simulink model "Simulink_Simulation"  (Simulink 10.1)
settings: Solver=ode23tb  StartTime=0.0  StopTime=3  RelTol=1e-3  EnableMultiTasking=on
undefined symbols (not defined in the file or in its folder): sigbuilder_block
libraries: powerlib x9, powerlib_meascontrol x1
settings Model: Creator=asus1  LastModifiedBy=x64
settings DataIOCC: LimitDataPoints=on
settings DebuggingCC: UnderspecifiedInitializationDetection=Simplified  MergeDetectMultiDrivingBlocksExec=error  SolverPrmCheckMsg=warning
settings GRTTargetCC: CombineOutputUpdateFcns=on  GRTInterface=off
settings ConfigComp: CovSFcnEnable=off
settings SimscapeCC: SimscapeNormalizeSystem=off

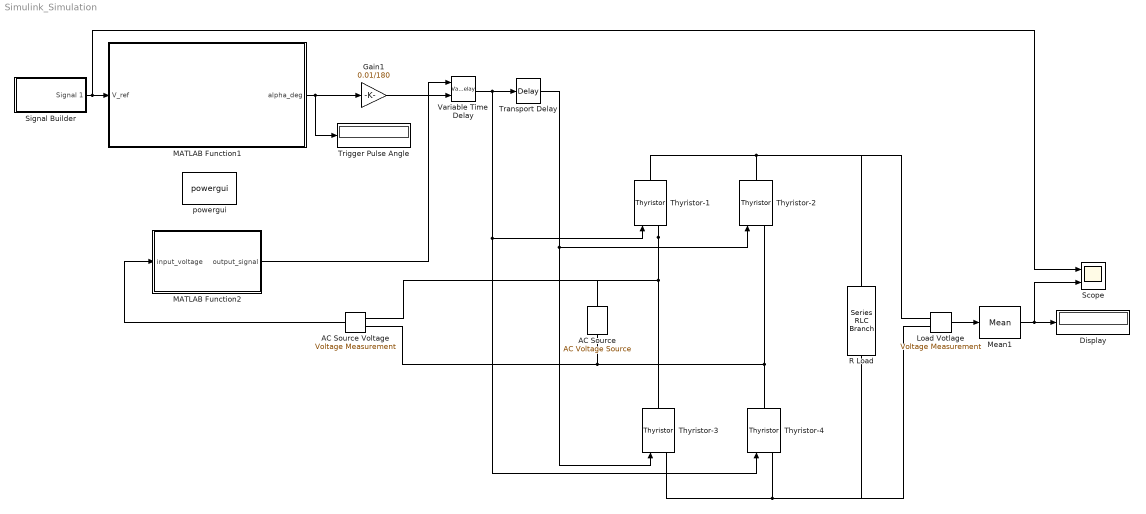
== system Simulink_Simulation ==
  AC Source : powerlib/Electrical Sources/AC Voltage Source  Amplitude=220*sqrt(2)  Phase=0  Frequency=50  SampleTime=0  Measurements=None  BusType=swing  Pref=10e3  Qref=0  Qmin=-inf  Qmax=+inf
  AC Source Voltage : powerlib/Measurements/Voltage Measurement  PhasorSimulation=off  OutputType=Complex  PSBequivalent=0
  "Display " : Display
  Gain1 : Gain  Gain=0.01/180
  Load Votlage : powerlib/Measurements/Voltage Measurement  PhasorSimulation=off  OutputType=Complex  PSBequivalent=0
  MATLAB Function1 : MATLAB Function  TreatAsAtomicUnit=on
  MATLAB Function2 : MATLAB Function  TreatAsAtomicUnit=on
  Mean1 : powerlib_meascontrol/Measurements/Mean  Freq=50  Vinit=0  Ts=0
  R Load : powerlib/Elements/Series RLC Branch  LConnTagsString=__new0  RConnTagsString=__new0  BranchType=R  Resistance=10  Inductance=1e-3  SetiL0=off  InitialCurrent=0  Capacitance=1e-6  Setx0=off  InitialVoltage=0  Measurements=None
  "Scope " : Scope  NumInputPorts=2
  "Signal Builder " : Subsystem  Tag=STV Subsys  LoadFcn=sigbuilder_block('load');  StartFcn=sigbuilder_block('start');  StopFcn=sigbuilder_block('stop');  ClipboardFcn=sigbuilder_block('clipboard');  mask(Sigbuilder block){tuvar=[0:10]}
      mask help: Simulink:masks:SigbuilderBlock_MD
      mask init:
      | if ~strcmp(get_param(bdroot(gcbh),'SimulationStatus'),'stopped') tuvar = sigbuilder_block('maskInit'); end
      settings: CopyFcn=sigbuilder_block('copy');  DeleteFcn=sigbuilder_block('delete');  ModelCloseFcn=sigbuilder_block('modelClose');  PreSaveFcn=sigbuilder_block('preSave');  PauseFcn=sigbuilder_block('pause');  ContinueFcn=sigbuilder_block('continue');  NameChangeFcn=sigbuilder_block('namechange');  OpenFcn=sigbuilder_block('open',[0 30 1152 561.6 ]);  CloseFcn=sigbuilder_block('close');
      mask Display: plot(0, 0, 100, 100,[2, 2, 32, 32, 2], [68, 8, 8, 68, 68],[32, 2], [38, 38], [32, 19, 2],[53, 60, 44], [32, 17, 17, 2],[16, 16, 31, 31]);txt = getActiveGroup(gcbh);text(2, 100, txt,'verticalAlignment', 'top');
  Thyristor-{1..4} (4 alike) : powerlib/Power Electronics/Thyristor  Ron=0.001  Lon=0  Vf=0.001  IC=0  Rs=1e5  Cs=inf  Measurements=off
  Transport Delay : TransportDelay  DelayTime=0.01
  Trigger Pulse Angle : Display
  Variable Time Delay : VariableTransportDelay  MaximumDelay=10
  powergui : powerlib/powergui  Priority=1  SimulationMode=Discrete  SampleTime=1e-6  frequency=60  Iterations=50  frequencyindice=50  Pbase=100e6  ErrMax=1e-4  UnitsV=kV  UnitsW=MW  buscounter=0  FunctionMessages=off  echomessages=off  EnableUseOfTLC=off  CurrentSourceSwitches=off  DisableSnubberDevices=off  DisableRonSwitches=off  DisableVfSwitches=off  DisplayEquations=off  AutomaticDiscreteSolvers=off  SolverType=Tustin  Interpol=off  ExternalGateDelay=off  methode=off  Ts=100  x0status=blocks  SPID=off  SwTol=0  HookPort=off  NonlinearTolerance=1e-4  nMaxIteration=100  ContinueOnMaxIteration=off  RestoreLinks=warning  ResistiveCurrentMeasurement=off  Frange=[0:2:500]  Ylog=off  Xlog=on  ShowGrid=off  save=off  variable=ZData  structure=0  ZoomFFT=off  StartTime=0.0  cycles=1  DisplayStyle=1  fundamental=60  FreqAxis=off  MaxFrequency=1000  frequencyindicesteady=1  RmsSteady=1  display=off
  wires:
  Transport Delay/1 -> Thyristor-3/1, Thyristor-2/1
  Variable Time Delay/1 -> Thyristor-4/1, Thyristor-1/1, Transport Delay/1
  Load Votlage/1 -> Mean1/1
  Mean1/1 -> "Display "/1, "Scope "/2
  "Signal Builder "/1(Signal 1) -> "Scope "/1, MATLAB Function1/1(V_ref)
  MATLAB Function1/1(alpha_deg) -> Gain1/1, Trigger Pulse Angle/1
  AC Source Voltage/1 -> MATLAB Function2/1(input_voltage)
  Gain1/1 -> Variable Time Delay/2
  MATLAB Function2/1(output_signal) -> Variable Time Delay/1
  connections:
  AC Source/LConn1 -- AC Source Voltage/LConn2 -- Thyristor-4/RConn1 -- Thyristor-2/LConn1
  Thyristor-1/LConn1 -- AC Source/RConn1 -- AC Source Voltage/LConn1 -- Thyristor-3/RConn1
  Thyristor-1/RConn1 -- Thyristor-2/RConn1 -- R Load/LConn1 -- Load Votlage/LConn1
  Thyristor-3/LConn1 -- Load Votlage/LConn2 -- R Load/RConn1 -- Thyristor-4/LConn1

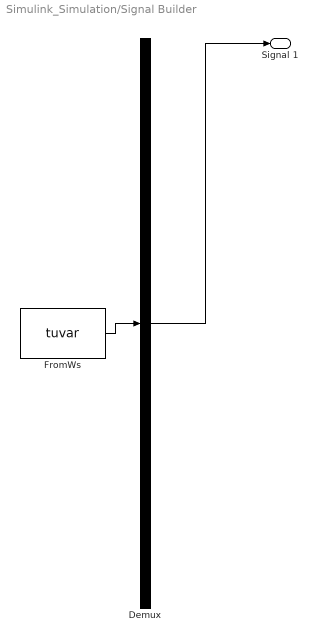
== system Simulink_Simulation/Signal Builder  ==
  Demux : Demux  Tag=STV Demux  Outputs=1
      settings: DisplayOption=none
  FromWs : FromWorkspace  Tag=STV FromWs  VariableName=tuvar  SigBuilderData=DataTag0  VnvData=DataTag1
      SigBuilderData=|
      | common.afterFinalStr = 'Extrapolate'
      | common.sampleTime = 0
      | dataSet.timeRange = [0 10]
      | dataSet.name = 'Group 1'
      | sbobj.Groups.Name = 'Group 1'
      | sbobj.Groups.Signals.Name = 'Signal 1'
      | sbobj.Groups.Signals.XData = [0 0.5 0.5 1 1 1.5 1.5 2 2 2.5 2.5 4 4 6 6 10]
      | sbobj.Groups.Signals.YData = [180 180 140 140 100 100 60 60 20 20 10 10 1 1 0 0]
  Signal 1 : Outport  Tag=STV Outport
  wires:
  Demux/1 -> Signal 1/1
  FromWs/1 -> Demux/1

== matlab function MATLAB Function1 ==
  data: V_ref input double; alpha_deg output double
function alpha_deg = Calculate_Alpha(V_ref)
    % Initialization of variables
    phi = 2;              % Initial guess for the angle (radians)
    eps_tol = 0.00001;    % Epsilon tolerance
    max_iter = 20;        % Maximum number of iterations
    diff_tol = 0.000001;  % Difference threshold
    alpha_deg = 0;        % Output angle initialization
    f_val = 0;            % Function value
    
    Vm = 220 * sqrt(2);   % Peak Voltage (Vm)
    
    % Newton-Raphson Loop
    for k = 1:max_iter
        % Derivative of the voltage equation: b = f'(phi)
        deriv = (Vm / pi) * sin(phi); 
        
        % Update rule: alpha = phi - f(phi)/f'(phi)
        % Equation being solved: V_ref - (Vm/pi)*(1 + cos(phi)) = 0
        numerator = -(Vm / pi) * (cos(phi) + 1) + V_ref;
        alpha_deg = phi - numerator / deriv;  
        
        % Error Calculation
        err_abs = abs(alpha_deg - phi);
        err_rel = 2 * err_abs / (abs(alpha_deg) + diff_tol);
        
        % Update phi for next step
        phi = alpha_deg;
        
        % Recalculate function residual
        f_val = -(Vm / pi) * (cos(phi) + 1) + V_ref;
        
        % Convergence Check
        if (err_abs < diff_tol) || (err_rel < diff_tol) || (abs(f_val) < eps_tol)
            break
        end 
    end
    
    % Convert result from Radians to Degrees
    alpha_deg = alpha_deg * 180 / pi;
end

== matlab function MATLAB Function2 ==
  data: output_signal output double; input_voltage input double
function output_signal = Zero_Crossing_Detector(input_voltage)
    % Checks if the input voltage is positive
    
    R = 10;             % Resistance (Ohm)
    epsilon = 0.000001; % Epsilon tolerance
    
    if input_voltage > 0
        output_signal = 1;
    else
        output_signal = 0;
    end
end
